simulink model "Boostcon"  (R2021a)
settings: Solver=VariableStepAuto  StartTime=0.0  StopTime=0.04  MaxStep=1e-6  RelTol=1e-3
values from neighbouring files (symbols this model uses):
  C = (Io*D*Ts)/deltaVo    (= 0.000514403292181)    [boost.m]
  D = 1-(Vg/Vo)    (= 0.333333333333)    [boost.m]
  L = (Vo*(1-D)*D*Ts)/delta_IL    (= 0.00018)    [boost.m]
  R = Vo^2/Po    (= 3.24)    [boost.m]
  Ts = 1/fs    (= 5e-05)    [boost.m]
  Vg = 12    [boost.m]
libraries: spsSeriesRLCBranchLib x5, spsCurrentMeasurementLib x3, spsBreakerLib x2, spsDCVoltageSourceLib x1, spsDiodeLib x1, spsGroundLib x1, spsMosfetLib x1, simulink x1, simulink_extras x1, spsVoltageMeasurementLib x1, spspowerguiLib x1
settings Model: Creator=mluser  LastModifiedBy=mluser

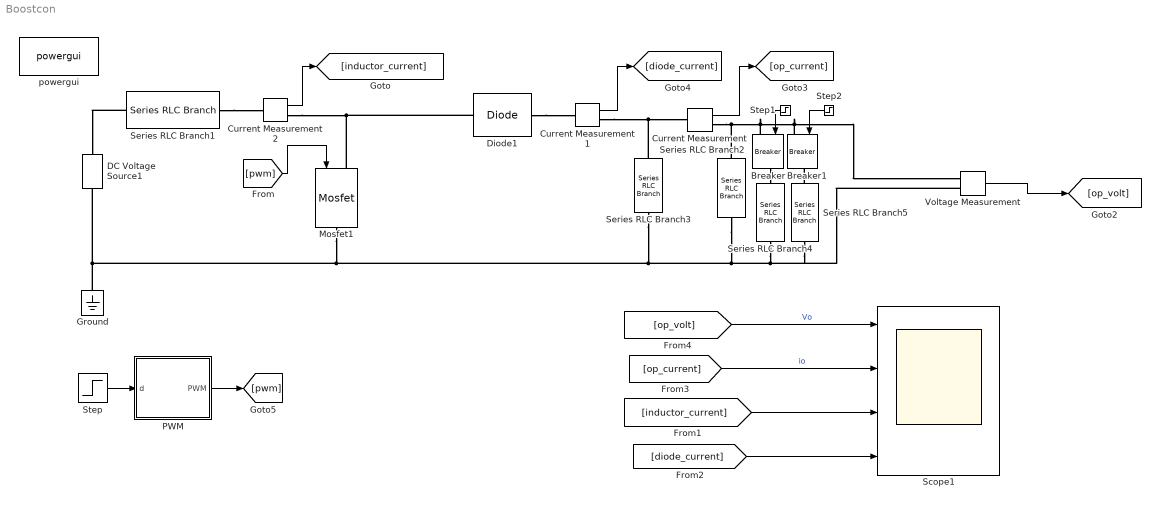
== system Boostcon ==
  Breaker : spsBreakerLib/Breaker  InitialState=0  SwitchingTimes="[1/60  5/60]"  External=on  BreakerResistance=0.01  SnubberResistance=1e6  SnubberCapacitance=inf  Measurements=None  MoreParameters=on  NoBreakLoop=off
      settings: SourceProductBaseCode=PS
  Breaker1 : spsBreakerLib/Breaker  InitialState=0  SwitchingTimes="[1/60  5/60]"  External=on  BreakerResistance=0.01  SnubberResistance=1e6  SnubberCapacitance=inf  Measurements=None  MoreParameters=on  NoBreakLoop=off
      settings: SourceProductBaseCode=PS
  Current Measurement : spsCurrentMeasurementLib/Current Measurement  PhasorSimulation=off  OutputType=Complex  PSBequivalent=0
  Current Measurement1 : spsCurrentMeasurementLib/Current Measurement  PhasorSimulation=off  OutputType=Complex  PSBequivalent=0
  Current Measurement2 : spsCurrentMeasurementLib/Current Measurement  PhasorSimulation=off  OutputType=Complex  PSBequivalent=0
  DC Voltage Source1 : spsDCVoltageSourceLib/DC Voltage Source  Amplitude=Vg  Measurements=None
  Diode1 : spsDiodeLib/Diode  Ron=0.001  Lon=0  Vf=0.8  IC=0  UseSnubber=0  Rs=inf  Cs=inf  Measurements=off
  Ground : spsGroundLib/Ground  LConnTagsString=a
  Mosfet1 : spsMosfetLib/Mosfet  Ron=0  Lon=0  Rd=0  Vfd=0  IC=0  Rs=1e5  Cs=inf  Measurements=off
  PWM : Subsystem
  Scope1 : Scope  NumInputPorts=4
  Series RLC Branch1 : spsSeriesRLCBranchLib/Series RLC Branch  LConnTagsString=__new0  RConnTagsString=__new0  BranchType=L  Resistance=1  Inductance=L  SetiL0=off  InitialCurrent=0  Capacitance=1e-6  Setx0=off  InitialVoltage=0  Measurements=None
  Series RLC Branch2 : spsSeriesRLCBranchLib/Series RLC Branch  LConnTagsString=__new0  RConnTagsString=__new0  BranchType=R  Resistance=R  Inductance=1e-3  SetiL0=off  InitialCurrent=0  Capacitance=1e-6  Setx0=off  InitialVoltage=0  Measurements=None
  Series RLC Branch3 : spsSeriesRLCBranchLib/Series RLC Branch  LConnTagsString=__new0  RConnTagsString=__new0  BranchType=C  Resistance=1  Inductance=1e-3  SetiL0=off  InitialCurrent=0  Capacitance=C  Setx0=off  InitialVoltage=0  Measurements=None
  Series RLC Branch4 : spsSeriesRLCBranchLib/Series RLC Branch  LConnTagsString=__new0  RConnTagsString=__new0  BranchType=R  Resistance=R  Inductance=1e-3  SetiL0=off  InitialCurrent=0  Capacitance=1e-6  Setx0=off  InitialVoltage=0  Measurements=None
  Series RLC Branch5 : spsSeriesRLCBranchLib/Series RLC Branch  LConnTagsString=__new0  RConnTagsString=__new0  BranchType=R  Resistance=4*R  Inductance=1e-3  SetiL0=off  InitialCurrent=0  Capacitance=1e-6  Setx0=off  InitialVoltage=0  Measurements=None
  Step : Step  Time=0.001  Before=D  After=D  SampleTime=0
  Step1 : Step  Time=0.02  SampleTime=0
  Step2 : Step  Time=0.032  SampleTime=0
  Voltage Measurement : spsVoltageMeasurementLib/Voltage Measurement  PhasorSimulation=off  OutputType=Complex  PSBequivalent=0
  powergui : spspowerguiLib/powergui  Priority=1  SimulationMode=Continuous  SampleTime=50e-6  frequency=60  Iterations=50  frequencyindice=0  Pbase=100e6  ErrMax=1e-4  UnitsV=kV  UnitsW=MW  buscounter=0  FunctionMessages=off  echomessages=off  EnableUseOfTLC=off  CurrentSourceSwitches=off  DisableSnubberDevices=off  DisableRonSwitches=off  DisableVfSwitches=off  DisplayEquations=off  AutomaticDiscreteSolvers=off  SolverType=Tustin/Backward Euler (TBE)  Interpol=off  ExternalGateDelay=off  methode=off  Ts=100  x0status=blocks  SPID=on  SwTol=0  HookPort=off  NonlinearTolerance=1e-4  nMaxIteration=100  ContinueOnMaxIteration=off  RestoreLinks=warning  ResistiveCurrentMeasurement=off  Frange=[0:2:500]  Ylog=off  Xlog=on  ShowGrid=off  save=off  variable=ZData  structure=0  ZoomFFT=off  StartTime=0.0  cycles=1  DisplayStyle=1  fundamental=60  FreqAxis=off  MaxFrequency=1000  frequencyindicesteady=1  RmsSteady=1  display=off
  wires:
  Current Measurement2/1 -> [inductor_current]
  Current Measurement1/1 -> [diode_current]
  Current Measurement/1 -> [op_current]
  Voltage Measurement/1 -> [op_volt]
  [inductor_current] -> Scope1/3
  [diode_current] -> Scope1/4
  [op_volt] -> Scope1/1  "Vo"
  Step/1 -> PWM/1(d)
  PWM/1(PWM) -> [pwm]
  [pwm] -> Mosfet1/1
  Step1/1 -> Breaker/1
  Step2/1 -> Breaker1/1
  [op_current] -> Scope1/2  "io"
  connections:
  Series RLC Branch1/LConn1 -- DC Voltage Source1/RConn1
  Current Measurement2/RConn1 -- Diode1/LConn1 -- Mosfet1/LConn1
  Series RLC Branch3/RConn1 -- Series RLC Branch5/RConn1 -- Voltage Measurement/LConn2 -- Series RLC Branch4/RConn1 -- Series RLC Branch2/RConn1 -- Mosfet1/RConn1 -- DC Voltage Source1/LConn1 -- Ground/LConn1
  Current Measurement/RConn1 -- Series RLC Branch2/LConn1 -- Breaker1/LConn1 -- Voltage Measurement/LConn1 -- Breaker/LConn1
  Current Measurement1/RConn1 -- Series RLC Branch3/LConn1 -- Current Measurement/LConn1
  Series RLC Branch1/RConn1 -- Current Measurement2/LConn1
  Diode1/RConn1 -- Current Measurement1/LConn1
  Breaker/RConn1 -- Series RLC Branch4/LConn1
  Series RLC Branch5/LConn1 -- Breaker1/RConn1

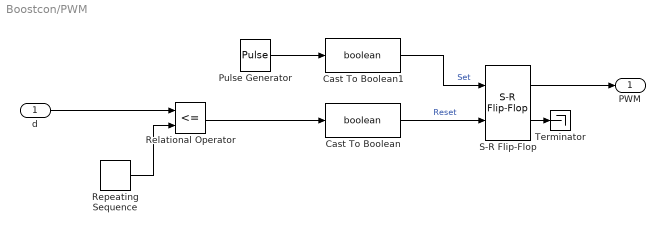
== system Boostcon/PWM ==
  d : Inport
  Cast To Boolean : DataTypeConversion  OutDataTypeStr=boolean
  Cast To Boolean1 : DataTypeConversion  OutDataTypeStr=boolean
  Pulse Generator : DiscretePulseGenerator  PulseType=Time based  Period=Ts  PulseWidth=5
  Relational Operator : RelationalOperator  Operator=<=  OutDataTypeStr=boolean  ZeroCross=off  RndMeth=Simplest
  Repeating Sequence : simulink/Sources/Repeating Sequence  rep_seq_t=[0 Ts]  rep_seq_y=[0 1]
  S-R Flip-Flop : simulink_extras/Flip Flops/S-R Flip-Flop  initial_condition=0
  Terminator : Terminator
  PWM : Outport
  wires:
  Repeating Sequence/1 -> Relational Operator/2
  Cast To Boolean/1 -> S-R Flip-Flop/2  "Reset"
  d/1 -> Relational Operator/1
  S-R Flip-Flop/1 -> PWM/1
  Pulse Generator/1 -> Cast To Boolean1/1
  S-R Flip-Flop/2 -> Terminator/1
  Cast To Boolean1/1 -> S-R Flip-Flop/1  "Set"
  Relational Operator/1 -> Cast To Boolean/1
